simulink model "double_feedback"  (R2015a)
settings: Solver=ode45  StartTime=0.0  StopTime=5  RelTol=1e-3
PreLoadFcn:
  | double_pend_feedback
InitFcn:
  | double_pend_feedback
StartFcn:
  | double_pend_feedback
values from neighbouring files (symbols this model uses):
  A = [zeros(3,3) eye(3); -inv(D_)*G zeros(3,3)]    [double_pend_feedback.m]    (also in fuzzy_logic.m = [zeros(3,3) eye(3); inv(D_)*G zeros(3,3)]; single_pend.m = [0 1 0 0; (g*(M+m))/(l*M) 0 0 b/(l*M); 0 0 0 1; -m*g/M 0 0 -)
  a = 0.1    [double_pend_feedback.m]    (also in fuzzy_logic.m; single_pend.m)
  A_ = [0 1 0 0; -k/mass -damper/mass (sqrt(ep*2*a*k))/ep*a*mass 0; 0 0 0 1; 0 0 0 -R/L]    [double_pend_feedback.m]    (also in fuzzy_logic.m; single_pend.m)
  B = [zeros(3,1); inv(D_)*H]    [double_pend_feedback.m]    (also in fuzzy_logic.m; single_pend.m = [0;-1/(l*M); 0 ; 1/M])
  B_ = [0; 1/mass; 0;0]    [double_pend_feedback.m]    (also in fuzzy_logic.m; single_pend.m)
  damper = 200    [double_pend_feedback.m]    (also in fuzzy_logic.m; single_pend.m)
  ep = 1    [double_pend_feedback.m]    (also in fuzzy_logic.m; single_pend.m)
  k = 1    [double_pend_feedback.m]    (also in fuzzy_logic.m; single_pend.m)
  K = double([sol.k1,sol.k2,sol.k3,sol.k4,sol.k5,sol.k6])    [double_pend_feedback.m]    (also in fuzzy_logic.m = lqr2; single_pend.m = [k1 k2 k3 k4])
  L = 0.0001    [double_pend_feedback.m]    (also in fuzzy_logic.m; single_pend.m)
  mass = 0.5    [double_pend_feedback.m]    (also in fuzzy_logic.m; single_pend.m)
  R = 100    [double_pend_feedback.m]    (also in fuzzy_logic.m; single_pend.m)
libraries: simulink x1
settings Model: Creator=Nabeel  LastModifiedBy=Nabeel

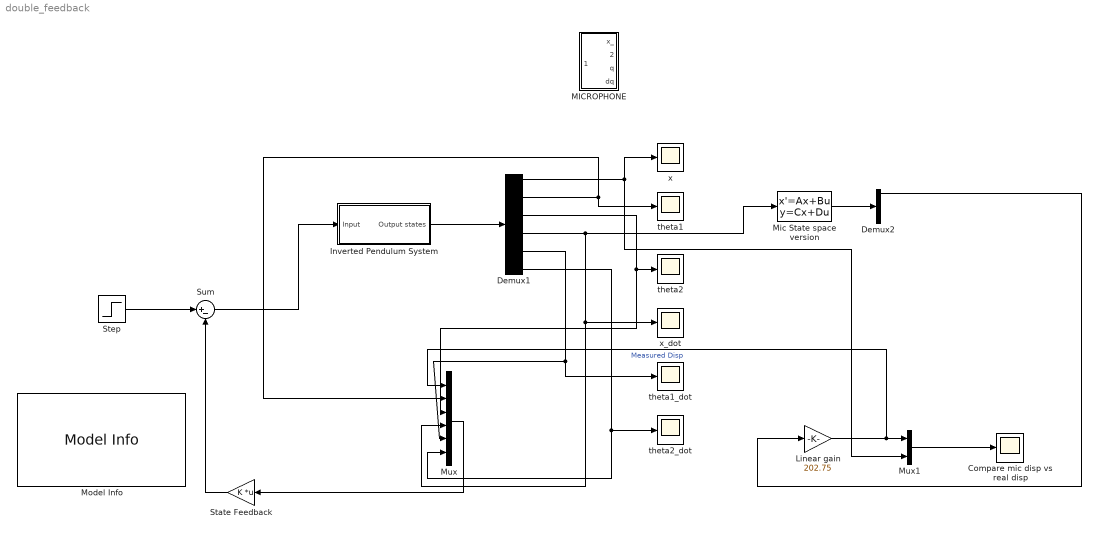
== system double_feedback ==
  Compare mic disp vs real disp : Scope
      settings: ShowLegends=on  SaveName=ScopeData24
  Demux1 : Demux  Outputs=6
  Demux2 : Demux
  Inverted Pendulum System : Subsystem
  Linear gain : Gain  Gain=202.75
  MICROPHONE : Subsystem
  Mic State space version : StateSpace  A=A_  B=B_  C=eye(4)  D=[0;0;0;0]  X0=0
  Model Info : simulink/Model-Wide Utilities/Model Info  Frame=on  DisplayStringWithTags=|  HorizontalTextAlignment=Center  LeftAlignmentValue=0.5  SourceBlockDiagram=double_feedback  TagMaxNumber=20
      | State feedback matrix info:
      | Replace the feedback block
      |  to test other controllers
      | Gain block
      | K- pole placement (non-repeated)
      | lqr1 - LQR 1 as defined in report
      | lqr2- LQR 2 as defined in the report
  Mux : Mux  Inputs=6
  Mux1 : Mux  Inputs=2
  State Feedback : Gain  Gain=K  Multiplication=Matrix(K*u)
  Step : Step  SampleTime=0
  Sum : Sum  Inputs=|+-
  theta1 : Scope
      settings: SaveName=theta1
  theta1_dot : Scope
      settings: SaveName=theta1_dot
  theta2 : Scope
      settings: SaveName=theta2
  theta2_dot : Scope
      settings: SaveName=theta2_dot
  x : Scope
      settings: SaveName=x
  x_dot : Scope
      settings: SaveName=x_dot
  wires:
  Step/1 -> Sum/1
  Inverted Pendulum System/1(Output states) -> Demux1/1
  Demux1/2 -> Mux/2, theta1/1
  Demux1/3 -> theta2/1, Mux/3
  Demux1/1 -> x/1, Mux1/2
  Mic State space version/1 -> Demux2/1
  Demux2/1 -> Linear gain/1
  Linear gain/1 -> Mux/1, Mux1/1  "Measured Disp"
  Mux1/1 -> Compare mic disp vs real disp/1
  Demux1/5 -> theta1_dot/1, Mux/5
  Demux1/6 -> theta2_dot/1, Mux/6
  State Feedback/1 -> Sum/2
  Sum/1 -> Inverted Pendulum System/1(Input)
  Demux1/4 -> Mic State space version/1, x_dot/1, Mux/4
  Mux/1 -> State Feedback/1

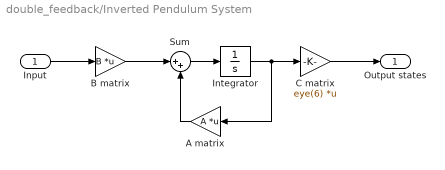
== system double_feedback/Inverted Pendulum System ==
  Input : Inport
  A matrix : Gain  Gain=A  Multiplication=Matrix(K*u)
  B matrix : Gain  Gain=B  Multiplication=Matrix(K*u)
  C matrix : Gain  Gain=eye(6)  Multiplication=Matrix(K*u)
  Integrator : Integrator  InitialCondition=[0 0 0 0 0 0]
  Sum : Sum  Inputs=|++
  Output states : Outport
  wires:
  Input/1 -> B matrix/1
  A matrix/1 -> Sum/2
  B matrix/1 -> Sum/1
  Sum/1 -> Integrator/1
  Integrator/1 -> C matrix/1, A matrix/1
  C matrix/1 -> Output states/1

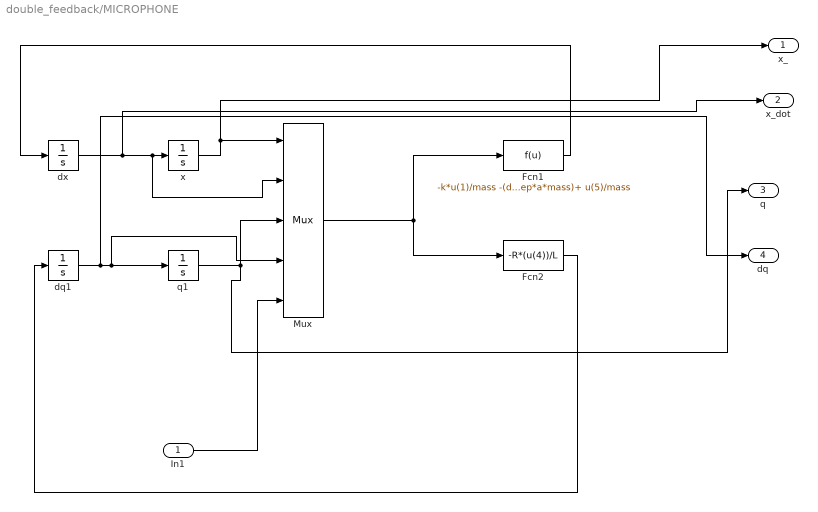
== system double_feedback/MICROPHONE ==
  In1 : Inport
  Fcn1 : Fcn  Expr=-k*u(1)/mass -(damper*u(2))/mass +(u(3))*((sqrt(ep*2*a*k))/ep*a*mass)+ u(5)/mass
  Fcn2 : Fcn  Expr=-R*(u(4))/L
  Mux : Mux  Inputs=5
  dq1 : Integrator
  dx : Integrator
  q1 : Integrator  InitialCondition=0.01  UpperSaturationLimit=3.14  LowerSaturationLimit=-3.14
  x : Integrator
  x_ : Outport
  x_dot : Outport  Port=2
  q : Outport  Port=3
  dq : Outport  Port=4
  wires:
  Fcn1/1 -> dx/1
  x/1 -> Mux/1, x_/1
  Mux/1 -> Fcn1/1, Fcn2/1
  q1/1 -> q/1, Mux/3
  Fcn2/1 -> dq1/1
  dq1/1 -> Mux/4, q1/1, dq/1
  dx/1 -> x_dot/1, Mux/2, x/1
  In1/1 -> Mux/5
